simulink model "Modulateur_AM"  (R2021a)
settings: Solver=VariableStepAuto  StartTime=0.0  StopTime=10.0  RelTol=1e-3
libraries: dspsrcs4 x1
settings Model: Creator=jimmypan  LastModifiedBy=jimmypan

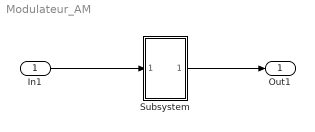
== system Modulateur_AM ==
  In1 : Inport
  Subsystem : Subsystem
  Out1 : Outport
  wires:
  In1/1 -> Subsystem/1(In1)
  Subsystem/1(Out1) -> Out1/1

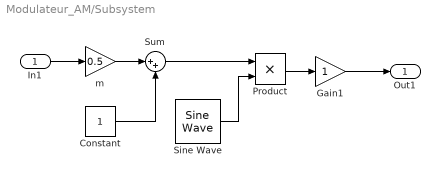
== system Modulateur_AM/Subsystem ==
  In1 : Inport
  Constant : Constant
  Gain1 : Gain
  Product : Product
  Sine Wave : dspsrcs4/Sine Wave  Amplitude=1  Frequency=20000  Phase=pi/2  SampleMode=Discrete  OutComplex=Real  CompMethod=Trigonometric fcn  TableSize=Speed  SampleTime=1/1000000  SamplesPerFrame=1  ResetState=Restart at time zero  OutputFrames=off  dataType=double  wordLen=16  udDataType=sfix(16)  fracBitsMode=Best precision  numFracBits=15  OutDataTypeStr=double  LastOutDataTypeStr=double
  Sum : Sum  Inputs=|++
  m : Gain  Gain=0.5
  Out1 : Outport
  wires:
  Sine Wave/1 -> Product/2
  Product/1 -> Gain1/1
  Gain1/1 -> Out1/1
  Sum/1 -> Product/1
  Constant/1 -> Sum/2
  In1/1 -> m/1
  m/1 -> Sum/1
